simulink model "Model4"  (R2020a)
settings: Solver=ode15s  StartTime=0.0  StopTime=70  RelTol=1e-3
values from neighbouring files (symbols this model uses):
  a = 1.2    [Init.m]
  a0 = 1.4    [Init.m]
  a1 = 0    [Init.m]
  a10 = 0    [Init.m]
  a11 = 0    [Init.m]
  a12 = 0    [Init.m]
  a13 = 0    [Init.m]
  a2 = 1100    [Init.m]
  a3 = 1100    [Init.m]
  a4 = 10    [Init.m]
  a5 = 0    [Init.m]
  a6 = 0    [Init.m]
  a7 = -2    [Init.m]
  a8 = 0    [Init.m]
  a9 = 0    [Init.m]
  alpha = 0.1    [vectarrow.m]
  Area = 2    [Init.m]
  b = 1.6    [Init.m]
  banking_indy = [0 0 0 0 0 0 0 0 0 0 0 0 ... (40234 elements, 1x40234)]    [banking_indy.mat]
  bankingON = 1    [Sim1.m]
  C_fuel = 0.0000003    (= 3e-07)    [Init.m]
  camber = 0    [Init.m]
  Cf = 100000    [Copy_of_LateralRegulatorProject.m]    (also in LatController.m; LateralControllerProject.m; LateralRegulatorProject.m; MoriSystem.m = 155000)
  Cr = 120000    [Copy_of_LateralRegulatorProject.m]    (also in LatController.m = 100000; LateralControllerProject.m = 100000; LateralRegulatorProject.m = 110000; MoriSystem.m = 205000)
  curveCenters = [    longStraight/2, curveCoord ... (first row only)    [track3d.m]
  Cx = 0.8    [Init.m]
  Cz = 1.5    [Init.m]
  errorThreshold = 15    [Controller.m]
  g = 9.81    [Init.m]
  init_vel = 20    [Init.m]    (also in Sim1.m)
  IT = 2875    [Init.m]
  K_wear = 10^(-9)    (= 1e-09)    [Init.m]
  l_f = 0.45    [Init.m]
  l_r = 0.55    [Init.m]
  longStraight = 1006    [track3d.m]
  lookahead = 30    [Controller.m]
  mT = 1500    [Init.m]    (also in VelRegulatorProject.m = 718)
  shortStraight = 201    [track3d.m]
  trajec = ones(5, size(s_curv, 2))    [RefTrajectory.m]    (also in RefTrajectory2.m)
  turn = 402.35    [track3d.m]
  Vx = 90    [Copy_of_LateralRegulatorProject.m]    (also in LatController.m = 70; LateralControllerProject.m = 55; LateralRegulatorProject.m = 70; MoriSystem.m = 16.6666666667)
undefined symbols (not defined in the file or in its folder): a14, a15, a16, a17, b1, b11, b12, b2, curvature_test, distanceThreshold, init_x_pos, init_yaw, m_fuel, overlapThreshold, rho_0, rho_1, slipstreamON, TyreContactAreaFront, TyreContactAreaRear, w1, w2
libraries: simulink x6
(part 2 of 2)

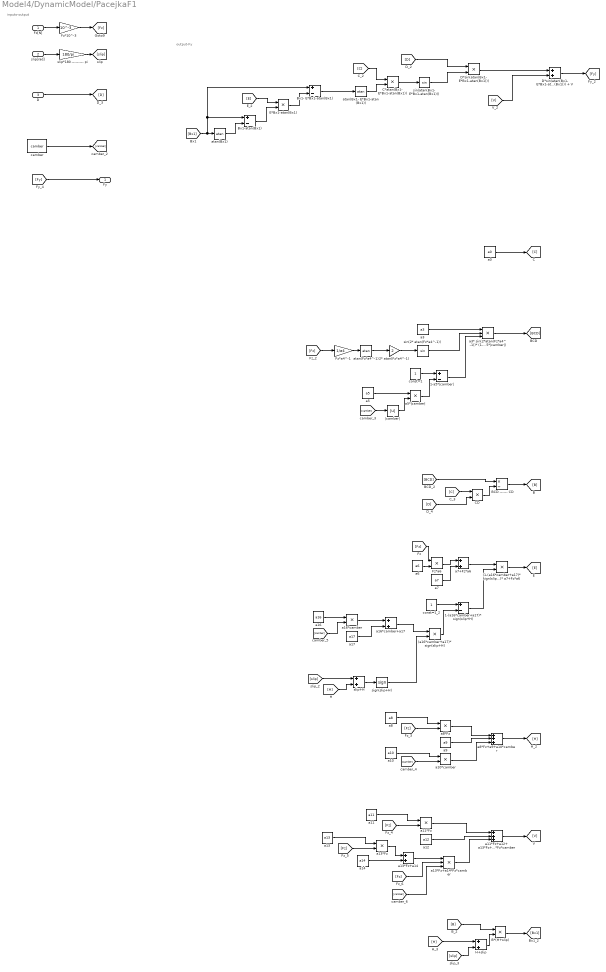
== system Model4/DynamicModel/PacejkaF1 ==
  note: inputs-output
  note: output-Fy
  Fz[N] : Inport  Unit=N
  slip[rad] : Inport  Port=2  Unit=rad
  D : Inport  Port=3
  (1-(a16*camber+a17)* sign(slip+H))* a7+Fz*a6 : Product
  (a16*camber+a17)* sign(slip+H) : Product
  1-(a16*camber+a17)* sign(slip+H) : Sum  Inputs=+-
  1-a5*|camber| : Sum  Inputs=+-
  2* atan(Fz*a4^-1) : Gain  Gain=2
  B*(H+slip) : Product
  BCD ------ CD : Product  Inputs=*/
  Bx1- E*Bx1-atan(Bx1) : Sum  Inputs=+-
  Bx1-atan(Bx1) : Sum  Inputs=+-
  C*atan(Bx1- E*Bx1-atan(Bx1)) : Product
  CD : Product
  D*sin(atan(Bx1- E*Bx1-atan(Bx1))) : Product
  D*sin(atan(Bx1- E*Bx1-atan(Bx1))) + V : Sum
  E*Bx1-atan(Bx1) : Product
  Fz*10^-3 : Gain  Gain=10^-3
  Fz*a4^-1 : Gain  Gain=1/a4
  Fz*a6 : Product
  H+slip : Sum
  a0 : Constant  Value=a0
  a10 : Constant  Value=a10
  a10*camber : Product
  a11 : Constant  Value=a11
  a11*Fz : Product
  a11*Fz+a12+ a13*Fz+a14*Fz*camber : Sum  Inputs=+++
  a12 : Constant  Value=a12
  a13 : Constant  Value=a13
  a13*Fz : Product
  a13*Fz+a14 : Sum
  a13*Fz+a14*Fz*camber : Product  Inputs=3
  a14 : Constant  Value=a14
  a16 : Constant  Value=a16
  a16*camber : Product
  a16*camber+a17 : Sum
  a17 : Constant  Value=a17
  a3 : Constant  Value=a3
  a3* sin(2*atan(Fz*a4^-1))* (1-a5*|camber|) : Product  Inputs=3
  a5 : Constant  Value=a5
  a5*|camber| : Product
  a6 : Constant  Value=a6
  a7 : Constant  Value=a7
  a7+Fz*a6 : Sum
  a8 : Constant  Value=a8
  a8*Fz : Product
  a8*Fz+a9+a10*camber : Sum  Inputs=+++
  a9 : Constant  Value=a9
  atan(Bx1) : Trigonometry  Operator=atan
  atan(Bx1- E*Bx1-atan(Bx1)) : Trigonometry  Operator=atan
  atan(Fz*a4^-1) : Trigonometry  Operator=atan
  camber : Constant  Value=camber
  const=1 : Constant
  const=1_2 : Constant
  sign(slip+H) : Signum  ZeroCross=off
  sin(2* atan(Fz*a4^-1)) : Trigonometry
  sin(atan(Bx1- E*Bx1-atan(Bx1))) : Trigonometry
  slip*180 --------- pi : Gain  Gain=180/pi
  slip+H : Sum
  |camber| : Abs
  Fy : Outport  Unit=N
  wires:
  C*atan(Bx1- E*Bx1-atan(Bx1))/1 -> sin(atan(Bx1- E*Bx1-atan(Bx1)))/1
  E*Bx1-atan(Bx1)/1 -> Bx1- E*Bx1-atan(Bx1)/2
  slip[rad]/1 -> slip*180 --------- pi/1
  1-a5*|camber|/1 -> a3* sin(2*atan(Fz*a4^-1))* (1-a5*|camber|)/3
  a10*camber/1 -> a8*Fz+a9+a10*camber/3
  |camber|/1 -> a5*|camber|/2
  a8/1 -> a8*Fz/1
  Fz*10^-3/1 -> [Fz]
  a0/1 -> [C]
  atan(Bx1- E*Bx1-atan(Bx1))/1 -> C*atan(Bx1- E*Bx1-atan(Bx1))/2
  [Fy] -> Fy/1
  Fz*a4^-1/1 -> atan(Fz*a4^-1)/1
  [B] -> B*(H+slip)/1
  [Fz] -> a8*Fz/2
  [Bx1] -> atan(Bx1)/1, Bx1-atan(Bx1)/1, Bx1- E*Bx1-atan(Bx1)/1
  [Fz] -> a13*Fz+a14*Fz*camber/2
  slip*180 --------- pi/1 -> [slip]
  2* atan(Fz*a4^-1)/1 -> sin(2* atan(Fz*a4^-1))/1
  [Fz] -> Fz*a6/1
  [slip] -> H+slip/2
  a11*Fz+a12+ a13*Fz+a14*Fz*camber/1 -> [V]
  a7+Fz*a6/1 -> (1-(a16*camber+a17)* sign(slip+H))* a7+Fz*a6/1
  [D] -> D*sin(atan(Bx1- E*Bx1-atan(Bx1)))/1
  a8*Fz+a9+a10*camber/1 -> [H]
  1-(a16*camber+a17)* sign(slip+H)/1 -> (1-(a16*camber+a17)* sign(slip+H))* a7+Fz*a6/2
  Bx1- E*Bx1-atan(Bx1)/1 -> atan(Bx1- E*Bx1-atan(Bx1))/1
  a3/1 -> a3* sin(2*atan(Fz*a4^-1))* (1-a5*|camber|)/1
  [camber] -> a16*camber/2
  [V] -> D*sin(atan(Bx1- E*Bx1-atan(Bx1))) + V/2
  [C] -> C*atan(Bx1- E*Bx1-atan(Bx1))/1
  B*(H+slip)/1 -> [Bx1]
  Fz[N]/1 -> Fz*10^-3/1
  camber/1 -> [camber]
  a11*Fz/1 -> a11*Fz+a12+ a13*Fz+a14*Fz*camber/1
  const=1/1 -> 1-a5*|camber|/1
  [Fz] -> a13*Fz/2
  a8*Fz/1 -> a8*Fz+a9+a10*camber/1
  [BCD] -> BCD ------ CD/1
  a14/1 -> a13*Fz+a14/2
  sin(atan(Bx1- E*Bx1-atan(Bx1)))/1 -> D*sin(atan(Bx1- E*Bx1-atan(Bx1)))/2
  sign(slip+H)/1 -> (a16*camber+a17)* sign(slip+H)/2
  a3* sin(2*atan(Fz*a4^-1))* (1-a5*|camber|)/1 -> [BCD]
  [camber] -> |camber|/1
  a13*Fz+a14/1 -> a13*Fz+a14*Fz*camber/1
  a9/1 -> a8*Fz+a9+a10*camber/2
  a16*camber/1 -> a16*camber+a17/1
  a12/1 -> a11*Fz+a12+ a13*Fz+a14*Fz*camber/2
  (1-(a16*camber+a17)* sign(slip+H))* a7+Fz*a6/1 -> [E]
  [Fz] -> Fz*a4^-1/1
  D*sin(atan(Bx1- E*Bx1-atan(Bx1))) + V/1 -> [Fy]
  BCD ------ CD/1 -> [B]
  a10/1 -> a10*camber/1
  [H] -> H+slip/1
  atan(Fz*a4^-1)/1 -> 2* atan(Fz*a4^-1)/1
  a16*camber+a17/1 -> (a16*camber+a17)* sign(slip+H)/1
  a11/1 -> a11*Fz/1
  a13*Fz/1 -> a13*Fz+a14/1
  a13*Fz+a14*Fz*camber/1 -> a11*Fz+a12+ a13*Fz+a14*Fz*camber/3
  a17/1 -> a16*camber+a17/2
  Fz*a6/1 -> a7+Fz*a6/1
  sin(2* atan(Fz*a4^-1))/1 -> a3* sin(2*atan(Fz*a4^-1))* (1-a5*|camber|)/2
  [Fz] -> a11*Fz/2
  [camber] -> a13*Fz+a14*Fz*camber/3
  Bx1-atan(Bx1)/1 -> E*Bx1-atan(Bx1)/2
  [C] -> CD/1
  [camber] -> a10*camber/2
  a6/1 -> Fz*a6/2
  [D] -> CD/2
  atan(Bx1)/1 -> Bx1-atan(Bx1)/2
  a13/1 -> a13*Fz/1
  (a16*camber+a17)* sign(slip+H)/1 -> 1-(a16*camber+a17)* sign(slip+H)/2
  D*sin(atan(Bx1- E*Bx1-atan(Bx1)))/1 -> D*sin(atan(Bx1- E*Bx1-atan(Bx1))) + V/1
  D/1 -> [D]
  H+slip/1 -> B*(H+slip)/2
  [E] -> E*Bx1-atan(Bx1)/1
  const=1_2/1 -> 1-(a16*camber+a17)* sign(slip+H)/1
  a7/1 -> a7+Fz*a6/2
  a16/1 -> a16*camber/1
  a5*|camber|/1 -> 1-a5*|camber|/2
  a5/1 -> a5*|camber|/1
  CD/1 -> BCD ------ CD/2
  [H] -> slip+H/2
  slip+H/1 -> sign(slip+H)/1
  [slip] -> slip+H/1

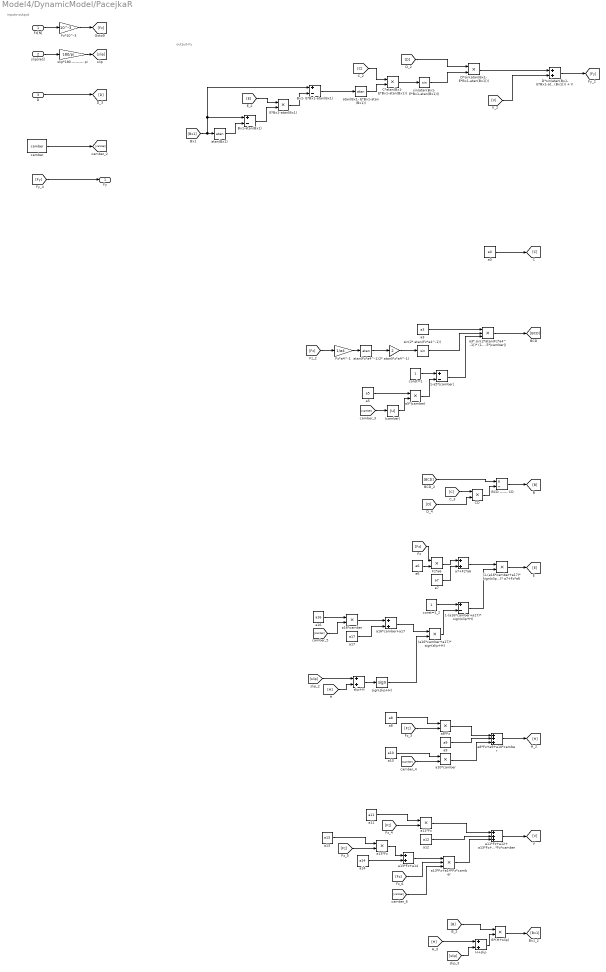
== system Model4/DynamicModel/PacejkaR ==
  note: inputs-output
  note: output-Fy
  Fz[N] : Inport  Unit=N
  slip[rad] : Inport  Port=2  Unit=rad
  D : Inport  Port=3
  (1-(a16*camber+a17)* sign(slip+H))* a7+Fz*a6 : Product
  (a16*camber+a17)* sign(slip+H) : Product
  1-(a16*camber+a17)* sign(slip+H) : Sum  Inputs=+-
  1-a5*|camber| : Sum  Inputs=+-
  2* atan(Fz*a4^-1) : Gain  Gain=2
  B*(H+slip) : Product
  BCD ------ CD : Product  Inputs=*/
  Bx1- E*Bx1-atan(Bx1) : Sum  Inputs=+-
  Bx1-atan(Bx1) : Sum  Inputs=+-
  C*atan(Bx1- E*Bx1-atan(Bx1)) : Product
  CD : Product
  D*sin(atan(Bx1- E*Bx1-atan(Bx1))) : Product
  D*sin(atan(Bx1- E*Bx1-atan(Bx1))) + V : Sum
  E*Bx1-atan(Bx1) : Product
  Fz*10^-3 : Gain  Gain=10^-3
  Fz*a4^-1 : Gain  Gain=1/a4
  Fz*a6 : Product
  H+slip : Sum
  a0 : Constant  Value=a0
  a10 : Constant  Value=a10
  a10*camber : Product
  a11 : Constant  Value=a11
  a11*Fz : Product
  a11*Fz+a12+ a13*Fz+a14*Fz*camber : Sum  Inputs=+++
  a12 : Constant  Value=a12
  a13 : Constant  Value=a13
  a13*Fz : Product
  a13*Fz+a14 : Sum
  a13*Fz+a14*Fz*camber : Product  Inputs=3
  a14 : Constant  Value=a14
  a16 : Constant  Value=a16
  a16*camber : Product
  a16*camber+a17 : Sum
  a17 : Constant  Value=a17
  a3 : Constant  Value=a3
  a3* sin(2*atan(Fz*a4^-1))* (1-a5*|camber|) : Product  Inputs=3
  a5 : Constant  Value=a5
  a5*|camber| : Product
  a6 : Constant  Value=a6
  a7 : Constant  Value=a7
  a7+Fz*a6 : Sum
  a8 : Constant  Value=a8
  a8*Fz : Product
  a8*Fz+a9+a10*camber : Sum  Inputs=+++
  a9 : Constant  Value=a9
  atan(Bx1) : Trigonometry  Operator=atan
  atan(Bx1- E*Bx1-atan(Bx1)) : Trigonometry  Operator=atan
  atan(Fz*a4^-1) : Trigonometry  Operator=atan
  camber : Constant  Value=camber
  const=1 : Constant
  const=1_2 : Constant
  sign(slip+H) : Signum  ZeroCross=off
  sin(2* atan(Fz*a4^-1)) : Trigonometry
  sin(atan(Bx1- E*Bx1-atan(Bx1))) : Trigonometry
  slip*180 --------- pi : Gain  Gain=180/pi
  slip+H : Sum
  |camber| : Abs
  Fy : Outport  Unit=N
  wires:
  C*atan(Bx1- E*Bx1-atan(Bx1))/1 -> sin(atan(Bx1- E*Bx1-atan(Bx1)))/1
  E*Bx1-atan(Bx1)/1 -> Bx1- E*Bx1-atan(Bx1)/2
  slip[rad]/1 -> slip*180 --------- pi/1
  1-a5*|camber|/1 -> a3* sin(2*atan(Fz*a4^-1))* (1-a5*|camber|)/3
  a10*camber/1 -> a8*Fz+a9+a10*camber/3
  |camber|/1 -> a5*|camber|/2
  a8/1 -> a8*Fz/1
  Fz*10^-3/1 -> [Fz]
  a0/1 -> [C]
  atan(Bx1- E*Bx1-atan(Bx1))/1 -> C*atan(Bx1- E*Bx1-atan(Bx1))/2
  [Fy] -> Fy/1
  Fz*a4^-1/1 -> atan(Fz*a4^-1)/1
  [B] -> B*(H+slip)/1
  [Fz] -> a8*Fz/2
  [Bx1] -> atan(Bx1)/1, Bx1-atan(Bx1)/1, Bx1- E*Bx1-atan(Bx1)/1
  [Fz] -> a13*Fz+a14*Fz*camber/2
  slip*180 --------- pi/1 -> [slip]
  2* atan(Fz*a4^-1)/1 -> sin(2* atan(Fz*a4^-1))/1
  [Fz] -> Fz*a6/1
  [slip] -> H+slip/2
  a11*Fz+a12+ a13*Fz+a14*Fz*camber/1 -> [V]
  a7+Fz*a6/1 -> (1-(a16*camber+a17)* sign(slip+H))* a7+Fz*a6/1
  [D] -> D*sin(atan(Bx1- E*Bx1-atan(Bx1)))/1
  a8*Fz+a9+a10*camber/1 -> [H]
  1-(a16*camber+a17)* sign(slip+H)/1 -> (1-(a16*camber+a17)* sign(slip+H))* a7+Fz*a6/2
  Bx1- E*Bx1-atan(Bx1)/1 -> atan(Bx1- E*Bx1-atan(Bx1))/1
  a3/1 -> a3* sin(2*atan(Fz*a4^-1))* (1-a5*|camber|)/1
  [camber] -> a16*camber/2
  [V] -> D*sin(atan(Bx1- E*Bx1-atan(Bx1))) + V/2
  [C] -> C*atan(Bx1- E*Bx1-atan(Bx1))/1
  B*(H+slip)/1 -> [Bx1]
  Fz[N]/1 -> Fz*10^-3/1
  camber/1 -> [camber]
  a11*Fz/1 -> a11*Fz+a12+ a13*Fz+a14*Fz*camber/1
  const=1/1 -> 1-a5*|camber|/1
  [Fz] -> a13*Fz/2
  a8*Fz/1 -> a8*Fz+a9+a10*camber/1
  [BCD] -> BCD ------ CD/1
  a14/1 -> a13*Fz+a14/2
  sin(atan(Bx1- E*Bx1-atan(Bx1)))/1 -> D*sin(atan(Bx1- E*Bx1-atan(Bx1)))/2
  sign(slip+H)/1 -> (a16*camber+a17)* sign(slip+H)/2
  a3* sin(2*atan(Fz*a4^-1))* (1-a5*|camber|)/1 -> [BCD]
  [camber] -> |camber|/1
  a13*Fz+a14/1 -> a13*Fz+a14*Fz*camber/1
  a9/1 -> a8*Fz+a9+a10*camber/2
  a16*camber/1 -> a16*camber+a17/1
  a12/1 -> a11*Fz+a12+ a13*Fz+a14*Fz*camber/2
  (1-(a16*camber+a17)* sign(slip+H))* a7+Fz*a6/1 -> [E]
  [Fz] -> Fz*a4^-1/1
  D*sin(atan(Bx1- E*Bx1-atan(Bx1))) + V/1 -> [Fy]
  BCD ------ CD/1 -> [B]
  a10/1 -> a10*camber/1
  [H] -> H+slip/1
  atan(Fz*a4^-1)/1 -> 2* atan(Fz*a4^-1)/1
  a16*camber+a17/1 -> (a16*camber+a17)* sign(slip+H)/1
  a11/1 -> a11*Fz/1
  a13*Fz/1 -> a13*Fz+a14/1
  a13*Fz+a14*Fz*camber/1 -> a11*Fz+a12+ a13*Fz+a14*Fz*camber/3
  a17/1 -> a16*camber+a17/2
  Fz*a6/1 -> a7+Fz*a6/1
  sin(2* atan(Fz*a4^-1))/1 -> a3* sin(2*atan(Fz*a4^-1))* (1-a5*|camber|)/2
  [Fz] -> a11*Fz/2
  [camber] -> a13*Fz+a14*Fz*camber/3
  Bx1-atan(Bx1)/1 -> E*Bx1-atan(Bx1)/2
  [C] -> CD/1
  [camber] -> a10*camber/2
  a6/1 -> Fz*a6/2
  [D] -> CD/2
  atan(Bx1)/1 -> Bx1-atan(Bx1)/2
  a13/1 -> a13*Fz/1
  (a16*camber+a17)* sign(slip+H)/1 -> 1-(a16*camber+a17)* sign(slip+H)/2
  D*sin(atan(Bx1- E*Bx1-atan(Bx1)))/1 -> D*sin(atan(Bx1- E*Bx1-atan(Bx1))) + V/1
  D/1 -> [D]
  H+slip/1 -> B*(H+slip)/2
  [E] -> E*Bx1-atan(Bx1)/1
  const=1_2/1 -> 1-(a16*camber+a17)* sign(slip+H)/1
  a7/1 -> a7+Fz*a6/2
  a16/1 -> a16*camber/1
  a5*|camber|/1 -> 1-a5*|camber|/2
  a5/1 -> a5*|camber|/1
  CD/1 -> BCD ------ CD/2
  [H] -> slip+H/2
  slip+H/1 -> sign(slip+H)/1
  [slip] -> slip+H/1

== matlab function Model4/Controller/prova2 ==
  data: x input; curvature output; y input; curveCenters input; longStraight input; shortStraight input; curve input; curvature_test input
function curvature = curvature2(x, y, curveCenters, ...
    longStraight, shortStraight, curve, curvature_test)

init_x = -271.4;
totL = 4023.4;
initD = pdist2([init_x, 0], [curveCenters(1,1),0]);

R = curve * 2 / pi;

% long straight 1
if y < curveCenters(1,2) && x >= curveCenters(4,1) && x <= curveCenters(1,1)
    d = pdist2([x, 0],[init_x, 0]);
    l = (totL - d)*(x < init_x) + ...
        (d)*(x >= init_x);
% long straight 2
elseif y > curveCenters(2,2) && x >= curveCenters(4,1) && x <= curveCenters(1,1)
    d = pdist2([x, 0],[curveCenters(2,1),0]);
    l = d + initD + shortStraight + 2*curve;
% short straigt 1
elseif x > 0 && y >= curveCenters(1,2) && y <= curveCenters(2,2)
    d = pdist2([y, 0],[curveCenters(1,2),0]);
    l = d + initD + curve;
% short straigt 2
elseif x < 0 && y >= curveCenters(1,2) && y <= curveCenters(2,2)
    d = pdist2([y, 0],[curveCenters(3,2),0]);
    l = d + initD + longStraight + shortStraight + 3*curve;
% curve 1
elseif x > curveCenters(1,1) && y < curveCenters(1,2)
    ang = asin((x - curveCenters(1,1))/pdist2([x,y],curveCenters(1,:)));
    l = ang * R + initD;
% curve 2
elseif x > curveCenters(2,1) && y > curveCenters(2,2)
    ang = asin((y - curveCenters(2,2))/pdist2([x,y],curveCenters(2,:)));
    l = ang * R + initD + curve + shortStraight;
% curve 3
elseif x < curveCenters(3,1) && y > curveCenters(3,2)
    ang = asin((-x + curveCenters(3,1))/pdist2([x,y],curveCenters(3,:)));
    l = ang * R + initD + curve*2 + shortStraight + longStraight;
% curve 4
elseif x < curveCenters(4,1) && y < curveCenters(4,2)
    ang = asin((-y + curveCenters(4,2))/pdist2([x,y],curveCenters(4,:)));
    l = ang * R + initD + curve*3 + shortStraight*2 + longStraight;
% default else
else 
    l = 0;
end

curvature = curvature_test(ceil(l*10),1);

== matlab function Model4/DynamicModel/yaw_ref ==
  data: egox input; egoy input; trajec input; ref output; cur_yaw input; index output; lookAhead input; errorThreshold input
function [ref,index] = yaw_ref(egox, egoy, trajec, cur_yaw, lookAhead, errorThreshold)%, curveCenters)

newEgox = egox + lookAhead*cos(cur_yaw);
newEgoy = egoy + lookAhead*sin(cur_yaw);

distArray = (newEgox - trajec(2,:)).^2 + (newEgoy - trajec(3,:)).^2;
[min_dist, real_index] = min(distArray);

min_dist = sqrt(min_dist);
index = real_index;

v1 = [newEgox - egox, newEgoy - egoy, 0];
v2 = [trajec(2, real_index) - egox, trajec(3, real_index) - egoy, 0];
C = cross(v1, v2);
if abs(C(3)) < errorThreshold
    ref = 0;
elseif sign(C(3)) == 1
    ref = -min_dist;
elseif sign(C(3)) == -1
    ref = min_dist;
else
    ref = 0;
end

% % long straight 1
% if newEgoy < curveCenters(1,2) && newEgox >= curveCenters(4,1) && newEgox <= curveCenters(1,1)
%     if newEgoy > -6.75 + threshold
%         ref = min_dist;
%     elseif newEgoy < -6.75 - threshold
%         ref = -min_dist;
%     else
%         ref = 0;
%     end
% % long straight 2
% elseif newEgoy > curveCenters(2,2) && newEgox >= curveCenters(4,1) && newEgox <= curveCenters(1,1)
%     if newEgoy < 720.04 - threshold
%         ref = min_dist;
%     elseif newEgoy > 720.04 + threshold
%         ref = -min_dist;
%     else
%         ref = 0;
%     end
% % short straigt 1
% elseif newEgox > 0 && newEgoy >= curveCenters(1,2) && newEgoy <= curveCenters(2,2)
%     if newEgox < 765.89 - threshold
%         ref = min_dist;
%     elseif newEgox > 765.89 + threshold
%         ref = -min_dist;
%     else
%         ref = 0;
%     end
% % short straigt 2
% elseif newEgox < 0 && newEgoy >= curveCenters(1,2) && newEgoy <= curveCenters(2,2)
%     if newEgox > -765.89 + threshold
%         ref = min_dist;
%     elseif newEgox < -765.89 - threshold
%         ref = -min_dist;
%     else
%         ref = 0;
%     end
% % curve 1
% elseif newEgox > curveCenters(1,1) && newEgoy < curveCenters(1,2)
%     myR = pdist2([newEgox,newEgoy],curveCenters(1,:));
%     trajR = pdist2([trajec(2, real_index),trajec(3, real_index)],curveCenters(1,:));
%     if myR > trajR + threshold
%         ref = -min_dist;
%     elseif myR < trajR - threshold
%         ref = min_dist;
%     else
%         ref = 0;
%     end
% % curve 2
% elseif newEgox > curveCenters(2,1) && newEgoy > curveCenters(2,2)
%     myR = pdist2([newEgox,newEgoy],curveCenters(2,:));
%     trajR = pdist2([trajec(2, real_index),trajec(3, real_index)],curveCenters(2,:));
%     if myR > trajR + threshold
%         ref = -min_dist;
%     elseif myR < trajR - threshold
%         ref = min_dist;
%     else
%         ref = 0;
%     end
% % curve 3
% elseif newEgox < curveCenters(3,1) && newEgoy > curveCenters(3,2)
%     myR = pdist2([newEgox,newEgoy],curveCenters(3,:));
%     trajR = pdist2([trajec(2, real_index),trajec(3, real_index)],curveCenters(3,:));
%     if myR > trajR + threshold
%         ref = -min_dist;
%     elseif myR < trajR - threshold
%         ref = min_dist;
%     else
%         ref = 0;
%     end
% % curve 4
% elseif newEgox < curveCenters(4,1) && newEgoy < curveCenters(4,2)
%     myR = pdist2([newEgox,newEgoy],curveCenters(4,:));
%     trajR = pdist2([trajec(2, real_index),trajec(3, real_index)],curveCenters(4,:));
%     if myR > trajR + threshold
%         ref = -min_dist;
%     elseif myR < trajR - threshold
%         ref = min_dist;
%     else
%         ref = 0;
%     end
% % default else
% else
%     ref = 0;
% end

== matlab function Model4/Controller/Longitudinal_controller/v_ref ==
  data: egox input; egoy input; trajec input; ref output
function ref = vel_ref(egox, egoy, trajec)

% index = floor(mod(pos*10, max_pos) + 1);
% thresh1 = 60;
% thresh2 = 20;
% from = max(1, index - thresh1);
% to = min(max_pos, index + thresh2);
% 
% real_index = from;
% min_dist = pdist2([trajec(2,real_index),trajec(3,real_index)],[egox, egoy]);
% for i=from+1:to
%     new_dist = pdist2([trajec(2,i),trajec(3,i)],[egox, egoy]);
%     if new_dist < min_dist
%         min_dist = new_dist;
%         real_index = i;
%     end
% end
distArray = (egox - trajec(2,:)).^2 + (egoy - trajec(3,:)).^2;
[~, real_index] = min(distArray);
ref = trajec(5, real_index);

% function ref = vel_ref(egox, egoy, trajec, cur_vel)
% 
% thresh = 5;
% maxp = 10;
% index = find( (abs(trajec(2,:) - egox) < thresh) & (abs(trajec(3,:) - egoy) < thresh), maxp);
% 
% if (isempty(index))
%     ref = cur_vel;
% else
%     
%     size_index = size(index, 2);
% 
%     real_index = index(1,1);
%     min_dist = pdist2([trajec(2,real_index),trajec(3,real_index)],[egox, egoy]);
% 
%     for i=2:size_index
%         new_dist = pdist2([trajec(2,index(1,i)),trajec(3,index(1,i))],[egox, egoy]);
%         if new_dist < min_dist
%             min_dist = new_dist;
%             real_index = index(1,i);
%         end
%     end
%     
%     ref = trajec(5, real_index);
% end

== matlab function Model4/DynamicModel/Banking ==
  data: x input; res output; y input; curveCenters input; longStraight input; shortStraight input; curve input; bankingON input; banking_indy input
function res = calculateBanking(x, y, curveCenters, ...
    longStraight, shortStraight, curve, ...
    bankingON, banking_indy)

% coder.extrinsic('evalin')
% coder.extrinsic('fitresult')
% fun = evalin('base','fitresult');

init_x = -271.4;
totL = 4023.4;
initD = pdist2([init_x, 0], [curveCenters(1,1),0]);

R = curve * 2 / pi;


if (bankingON < 1)
    res = 0;
else
    % long straight 1
    if y < curveCenters(1,2) && x >= curveCenters(4,1) && x <= curveCenters(1,1)
        d = pdist2([x, 0],[init_x, 0]);
        l = (totL - d)*(x < init_x) + ...
            (d)*(x >= init_x);
    % long straight 2
    elseif y > curveCenters(2,2) && x >= curveCenters(4,1) && x <= curveCenters(1,1)
        d = pdist2([x, 0],[curveCenters(2,1),0]);
        l = d + initD + shortStraight + 2*curve;
    % short straigt 1
    elseif x > 0 && y >= curveCenters(1,2) && y <= curveCenters(2,2)
        d = pdist2([y, 0],[curveCenters(1,2),0]);
        l = d + initD + curve;
    % short straigt 2
    elseif x < 0 && y >= curveCenters(1,2) && y <= curveCenters(2,2)
        d = pdist2([y, 0],[curveCenters(3,2),0]);
        l = d + initD + longStraight + shortStraight + 3*curve;
    % curve 1
    elseif x > curveCenters(1,1) && y < curveCenters(1,2)
        ang = asin((x - curveCenters(1,1))/pdist2([x,y],curveCenters(1,:)));
        l = ang * R + initD;
    % curve 2
    elseif x > curveCenters(2,1) && y > curveCenters(2,2)
        ang = asin((y - curveCenters(2,2))/pdist2([x,y],curveCenters(2,:)));
        l = ang * R + initD + curve + shortStraight;
    % curve 3
    elseif x < curveCenters(3,1) && y > curveCenters(3,2)
        ang = asin((-x + curveCenters(3,1))/pdist2([x,y],curveCenters(3,:)));
        l = ang * R + initD + curve*2 + shortStraight + longStraight;
    % curve 4
    elseif x < curveCenters(4,1) && y < curveCenters(4,2)
        ang = asin((-y + curveCenters(4,2))/pdist2([x,y],curveCenters(4,:)));
        l = ang * R + initD + curve*3 + shortStraight*2 + longStraight;
    % default else
    else 
        l = 0;
    end
    
    %res = fun(l);
    res = banking_indy(ceil(l*10),1);
    %res = 0;
end

% function res = calculateBanking(x, y, curveCenters, ...
%     bankingThresholdLong, bankingThresholdShort, bankingAngle, midY, ...
%     bankingON)
% if (bankingON < 1)
%     res = 0;
% else
%     if(y < curveCenters(1,2) || y > curveCenters(2,2)) 
%        if(abs(x) < curveCenters(1,1) - bankingThresholdLong)
%            res = 0;
%        elseif (abs(x) > curveCenters(1,1))
%            res = bankingAngle;
%        else
%            res = bankingAngle*( 1 - ((abs(x) -  curveCenters(1,1))/(-bankingThresholdLong)) );
%        end
%     else
%         if (abs(y-midY) < curveCenters(2,2) - bankingThresholdShort - midY)
%             res = 0;
%         else
%             res = bankingAngle*( 1 - ((abs(y-midY) -  curveCenters(2,2) + midY)/(-bankingThresholdShort)) );
%         end
%     end
% end

== matlab function Model4/Controller/prova ==
  data: egox input; egoy input; curveCenters input; curvature output; trajec input; vel_ref output; error output; cur_yaw input; b input
function [curvature, vel_ref, error] = curv(egox, egoy, curveCenters, trajec, cur_yaw, b)

rearEgox = egox - b*cos(cur_yaw);
rearEgoy = egoy - b*sin(cur_yaw);

distArray = (rearEgox - trajec(2,:)).^2 + (rearEgoy - trajec(3,:)).^2;
% distArray = (egox - trajec(2,:)).^2 + (egoy - trajec(3,:)).^2;
[min_dist, real_index] = min(distArray);
min_dist = sqrt(min_dist);
v1 = [egox - egox + b*cos(cur_yaw), egoy - egoy + b*sin(cur_yaw), 0];
v2 = [trajec(2, real_index) - egox, trajec(3, real_index) - egoy, 0];
C = cross(v1, v2);
if sign(C(3)) == 1
    error = -min_dist;
elseif sign(C(3)) == -1
    error = min_dist;
else
    error = 0;
end

deltaS = 10;
indexLookahead = real_index + floor(deltaS * 10);
if indexLookahead > size(trajec, 2)
   indexLookahead = indexLookahead - size(trajec, 2);
end
lookaheadPoint = [trajec(2, indexLookahead), trajec(3, indexLookahead)];
ld = pdist2([rearEgox, rearEgoy], lookaheadPoint);

x0_1 = rearEgox;
x1_1 = rearEgox + cos(cur_yaw);
y0_1 = rearEgoy;
y1_1 = rearEgoy + sin(cur_yaw);
m1 = (y1_1-y0_1)/(x1_1-x0_1);
% k1 = -m*x0_1+y0_1;

x0_2 = rearEgox;
x1_2 = lookaheadPoint(1);
y0_2 = rearEgoy;
y1_2 = lookaheadPoint(2);
m2 = (y1_2-y0_2)/(x1_2-x0_2);
% k2 = -m*x0_2+y0_2;

alfa_t = atan((m1-m2)/(1+m1*m2));
curvature = sign(C(3))*2*sin(alfa_t)/ld;

% % long straight 1
% if egoy < curveCenters(1,2) && egox >= curveCenters(4,1) && egox <= curveCenters(1,1)
%     curvature = 0;
% % long straight 2
% elseif egoy > curveCenters(2,2) && egox >= curveCenters(4,1) && egox <= curveCenters(1,1)
%     curvature = 0;
% % short straigt 1
% elseif egox > 0 && egoy >= curveCenters(1,2) && egoy <= curveCenters(2,2)
%     curvature = 0;
% % short straigt 2
% elseif egox < 0 && egoy >= curveCenters(1,2) && egoy <= curveCenters(2,2)
%     curvature = 0;
% % curve 1
% elseif egox > curveCenters(1,1) && egoy < curveCenters(1,2)
%     Rcurv = pdist2([trajec(2,real_index), trajec(3, real_index)],curveCenters(1,:));
%     curvature = 1/Rcurv;
% % curve 2
% elseif egox > curveCenters(2,1) && egoy > curveCenters(2,2)
%     Rcurv = pdist2([trajec(2,real_index), trajec(3, real_index)],curveCenters(2,:));
%     curvature = 1/Rcurv;
% % curve 3
% elseif egox < curveCenters(3,1) && egoy > curveCenters(3,2)
%     Rcurv = pdist2([trajec(2,real_index), trajec(3, real_index)],curveCenters(3,:));
%     curvature = 1/Rcurv;
% % curve 4
% elseif egox < curveCenters(4,1) && egoy < curveCenters(4,2)
%     Rcurv = pdist2([trajec(2,real_index), trajec(3, real_index)],curveCenters(4,:));
%     curvature = 1/Rcurv;
% % default else
% else
%     curvature = 0;
% end

vel_ref = trajec(5, real_index);

== matlab function Model4/DynamicModel/periodic ==
  data: yaw input; periodicYaw output
function periodicYaw = periodic(yaw)

periodicYaw = abs(yaw) - (2*pi * floor(abs(yaw)/(2*pi)));

== matlab function Model4/DynamicModel/WindEffect ==
  data: rho_0 input; aerodynamic_coeff output; rho_1 input; ego_x input; ego_y input; opp_x input; opp_y input; distanceThreshold input; overlapThreshold input; alpha input; curveCenters input; slipstreamON input
function aerodynamic_coeff = windEffect(rho_0, rho_1, ego_x, ego_y, ... 
    opp_x, opp_y, distanceThreshold, overlapThreshold, alpha, curveCenters, ...
    slipstreamON)

if(slipstreamON < 1)
    aerodynamic_coeff = rho_0;
else
    %give in output rho_0 if too distant from other vehicle
    %rho_1 otherwise
    distanceThresholdCurve =  alpha * distanceThreshold;
    overlapThresholdCurve =  alpha * overlapThreshold;

    if  ego_x > curveCenters(1,1) && ego_y < curveCenters(1,2) %check if in the first curve
        ego_radius = sqrt((ego_x - curveCenters(1,1))^2 + (ego_y - curveCenters(1,2))^2);
        opp_radius = sqrt((opp_x - curveCenters(1,1))^2 + (opp_y - curveCenters(1,2))^2);
        if abs(ego_radius - opp_radius) < overlapThresholdCurve && ...
                sqrt((ego_x - opp_x)^2 + (ego_y - opp_y)^2) < distanceThresholdCurve && ...
                ego_y < opp_y
            aerodynamic_coeff = rho_1;
        else
           aerodynamic_coeff = rho_0;
        end
    elseif ego_x > curveCenters(2,1) && ego_y > curveCenters(2,2) %check if in the second curve
        ego_radius = sqrt((ego_x - curveCenters(2,1))^2 + (ego_y - curveCenters(2,2))^2);
        opp_radius = sqrt((opp_x - curveCenters(2,1))^2 + (opp_y - curveCenters(2,2))^2);
        if abs(ego_radius - opp_radius) < overlapThresholdCurve && ...
                sqrt((ego_x - opp_x)^2 + (ego_y - opp_y)^2) < distanceThresholdCurve && ...
                ego_x > opp_x
            aerodynamic_coeff = rho_1;
        else
           aerodynamic_coeff = rho_0;
        end
    elseif ego_x < curveCenters(3,1) && ego_y > curveCenters(3,2) %check if in the third curve
        ego_radius = sqrt((ego_x - curveCenters(3,1))^2 + (ego_y - curveCenters(3,2))^2);
        opp_radius = sqrt((opp_x - curveCenters(3,1))^2 + (opp_y - curveCenters(3,2))^2);
        if abs(ego_radius - opp_radius) < overlapThresholdCurve && ...
                sqrt((ego_x - opp_x)^2 + (ego_y - opp_y)^2) < distanceThresholdCurve && ...
                ego_y > opp_y
            aerodynamic_coeff = rho_1;
        else
           aerodynamic_coeff = rho_0;
        end
    elseif ego_x < curveCenters(4,1) && ego_y < curveCenters(4,2) %check if in the fourth curve
        ego_radius = sqrt((ego_x - curveCenters(4,1))^2 + (ego_y - curveCenters(4,2))^2);
        opp_radius = sqrt((opp_x - curveCenters(4,1))^2 + (opp_y - curveCenters(4,2))^2);
        if abs(ego_radius - opp_radius) < overlapThresholdCurve && ...
                sqrt((ego_x - opp_x)^2 + (ego_y - opp_y)^2) < distanceThresholdCurve && ...
                ego_x < opp_x
            aerodynamic_coeff = rho_1;
        else
           aerodynamic_coeff = rho_0;
        end
    else
        %check for which straights
        if ego_y < curveCenters(1,2) && ego_x >= curveCenters(4,1) && ego_x <= curveCenters(1,1)
           %first long straight
           if abs(ego_y - opp_y) < overlapThreshold && ...
                   abs(opp_x - ego_x) < distanceThreshold && ...
                   ego_x < opp_x
               aerodynamic_coeff = rho_1;
           else
               aerodynamic_coeff = rho_0;
           end

        elseif ego_y > curveCenters(2,2) && ego_x >= curveCenters(3,1) && ego_x <= curveCenters(2,1)
           %second long straight
           if abs(ego_y - opp_y) < overlapThreshold && ...
                   abs(opp_x - ego_x) < distanceThreshold && ...
                   ego_x > opp_x
               aerodynamic_coeff = rho_1;
           else
               aerodynamic_coeff = rho_0;
           end

        elseif ego_x > curveCenters(1,1) && ego_y >= curveCenters(1,2) && ego_y <= curveCenters(2,2)
           %first short straight
           if abs(ego_x - opp_x) < overlapThreshold && ...
                   abs(opp_y - ego_y) < distanceThreshold && ...
                   ego_y < opp_y
               aerodynamic_coeff = rho_1;
           else
               aerodynamic_coeff = rho_0;
           end

        elseif ego_x < curveCenters(3,1) && ego_y >= curveCenters(4,2) && ego_y <= curveCenters(3,2)
           %second short straight
           if abs(ego_x - opp_x) < overlapThreshold && ...
                   abs(opp_y - ego_y) < distanceThreshold && ...
                   ego_y > opp_y
               aerodynamic_coeff = rho_1;
           else
               aerodynamic_coeff = rho_0;
           end

        else
            aerodynamic_coeff = rho_0;
        end
    end
end
